simulink model "WPT_1"  (R2024a)
settings: Solver=VariableStepAuto  StartTime=0.0  StopTime=5  RelTol=1e-3
libraries: spsDiodeLib x9, spsSeriesRLCBranchLib x7, spsMosfetLib x5, spsVoltageMeasurementLib x4, spsCurrentMeasurementLib x3, spsMeanLib x3, spsACVoltageSourceLib x1, spsMutualInductanceLib x1, sps_lib x1
settings Model: Creator=Vivek Chadgal  LastModifiedBy=Vivek Chadgal
settings SolverCC: ZeroCrossAlgorithm=Adaptive
settings DebuggingCC: IgnoredZcDiagnostic=none

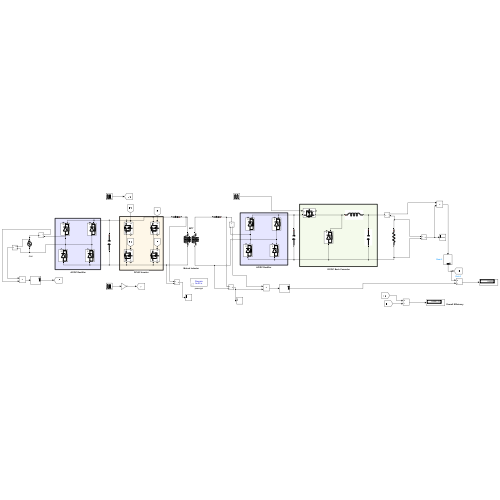
[thumbnail: Simulink's stored preview of the top-level diagram]
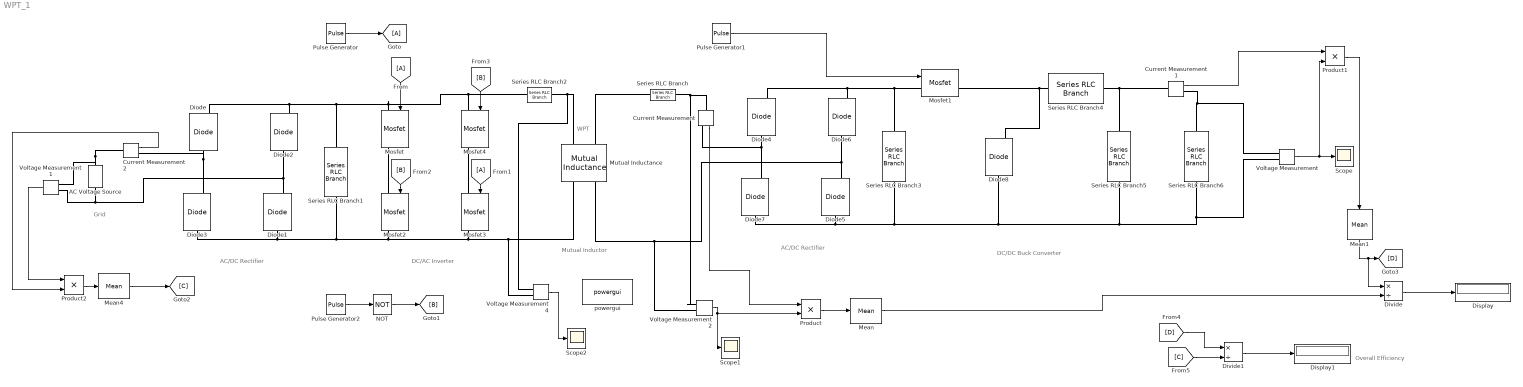
== system WPT_1 ==
  note: Overall Efficiency
  note: WPT
  note: Mutual Inductor
  note: Grid
  note: AC/DC Rectifier
  note: DC/DC Buck Converter
  note: DC/AC Inverter
  note: AC/DC Rectifier
  AC Voltage Source : spsACVoltageSourceLib/AC Voltage Source  Amplitude=230  Phase=0  Frequency=50  SampleTime=0  Measurements=None  BusType=swing  Pref=10e3  Qref=0  Qmin=-inf  Qmax=+inf
  Current Measurement : spsCurrentMeasurementLib/Current Measurement  PhasorSimulation=off  OutputType=Complex  PSBequivalent=0
  Current Measurement1 : spsCurrentMeasurementLib/Current Measurement  PhasorSimulation=off  OutputType=Complex  PSBequivalent=0
  Current Measurement2 : spsCurrentMeasurementLib/Current Measurement  PhasorSimulation=off  OutputType=Complex  PSBequivalent=0
  Diode{,1..8} (9 alike) : spsDiodeLib/Diode  Ron=0.001  Lon=0  Vf=0.8  IC=0  UseSnubber=0  Rs=500  Cs=250e-9  Measurements=on
  Display : Display
  Display1 : Display
  Divide : Product  Inputs=*/
  Divide1 : Product  Inputs=*/
  From : From
  From1 : From
  Goto : Goto
  Mean : spsMeanLib/Mean  Freq=50  Vinit=0  Ts=0
  Mean1 : spsMeanLib/Mean  Freq=50  Vinit=0  Ts=0
  Mean4 : spsMeanLib/Mean  Freq=50  Vinit=0  Ts=0
  Mosfet{,1..4} (5 alike) : spsMosfetLib/Mosfet  Ron=0.1  Lon=0  Rd=0.01  Vfd=0  IC=0  Rs=1e5  Cs=inf  Measurements=on
  Mutual Inductance : spsMutualInductanceLib/Mutual Inductance  LConnTagsString=a|b  RConnTagsString=A|B  TypeOfMutual=Two or three windings with equal mutual terms  NumberOfWindings=2  SelfImpedance1=[0 0.25]  SelfImpedance2=[ 0 0.25]  ThreeWindings=off  SelfImpedance3=[ 1.1 1.1e-03]  MutualImpedance=[0 0.125]  InductanceMatrix="[1.0 0.9  0.9 ;  0.9 1.0  0.9;  0.9 0.9 1.0 ] * 1e-3"  ResistanceMatrix="[1.0 0.9  0.9 ;  0.9 1.0  0.9;  0.9 0.9 1.0 ]"  Measurements=Winding voltages and currents
      settings: LibrarySourceBlock=sps_lib/Passives/Mutual Inductance
  NOT : Logic  Operator=NOT  IconShape=distinctive  AllPortsSameDT=off  OutDataTypeStr=boolean
  Product : Product
  Product1 : Product
  Product2 : Product
  Pulse Generator : DiscretePulseGenerator  PulseType=Time based  Amplitude=5  Period=0.02  PulseWidth=50
  Pulse Generator1 : DiscretePulseGenerator  PulseType=Time based  Amplitude=5  Period=0.02  PulseWidth=50
  Pulse Generator2 : DiscretePulseGenerator  PulseType=Time based  Amplitude=50  Period=0.02  PulseWidth=5
  Scope : Scope
  Scope1 : Scope
  Scope2 : Scope
  Series RLC Branch : spsSeriesRLCBranchLib/Series RLC Branch  LConnTagsString=__new0  RConnTagsString=__new0  BranchType=C  Resistance=1  Inductance=1e-3  SetiL0=off  InitialCurrent=0  Capacitance=4.691e-6  Setx0=off  InitialVoltage=0  Measurements=None
  Series RLC Branch1 : spsSeriesRLCBranchLib/Series RLC Branch  LConnTagsString=__new0  RConnTagsString=__new0  BranchType=C  Resistance=1  Inductance=1e-3  SetiL0=off  InitialCurrent=0  Capacitance=10e-6  Setx0=off  InitialVoltage=0  Measurements=None
  Series RLC Branch2 : spsSeriesRLCBranchLib/Series RLC Branch  LConnTagsString=__new0  RConnTagsString=__new0  BranchType=C  Resistance=1  Inductance=1e-3  SetiL0=off  InitialCurrent=0  Capacitance=4.691e-6  Setx0=off  InitialVoltage=0  Measurements=None
  Series RLC Branch3 : spsSeriesRLCBranchLib/Series RLC Branch  LConnTagsString=__new0  RConnTagsString=__new0  BranchType=C  Resistance=1  Inductance=1e-3  SetiL0=off  InitialCurrent=0  Capacitance=1000e-6  Setx0=off  InitialVoltage=0  Measurements=None
  Series RLC Branch4 : spsSeriesRLCBranchLib/Series RLC Branch  LConnTagsString=__new0  RConnTagsString=__new0  BranchType=L  Resistance=1  Inductance=1e-3  SetiL0=off  InitialCurrent=0  Capacitance=1e-6  Setx0=off  InitialVoltage=0  Measurements=None
  Series RLC Branch5 : spsSeriesRLCBranchLib/Series RLC Branch  LConnTagsString=__new0  RConnTagsString=__new0  BranchType=C  Resistance=1  Inductance=1e-3  SetiL0=off  InitialCurrent=0  Capacitance=1000e-6  Setx0=off  InitialVoltage=0  Measurements=None
  Series RLC Branch6 : spsSeriesRLCBranchLib/Series RLC Branch  LConnTagsString=__new0  RConnTagsString=__new0  BranchType=R  Resistance=1000  Inductance=1e-3  SetiL0=off  InitialCurrent=0  Capacitance=1e-6  Setx0=off  InitialVoltage=0  Measurements=None
  Voltage Measurement{,1..2,4} (4 alike) : spsVoltageMeasurementLib/Voltage Measurement  PhasorSimulation=off  OutputType=Complex  PSBequivalent=0
  powergui : sps_lib/powergui  Priority=1  SimulationMode=Discrete  SampleTime=50e-6  frequency=60  Iterations=50  frequencyindice=50  Pbase=100e6  ErrMax=1e-4  UnitsV=kV  UnitsW=MW  buscounter=0  FunctionMessages=off  echomessages=off  EnableUseOfTLC=off  CurrentSourceSwitches=off  DisableSnubberDevices=off  DisableRonSwitches=off  DisableVfSwitches=off  DisplayEquations=off  AutomaticDiscreteSolvers=off  SolverType=Tustin/Backward Euler (TBE)  Interpol=off  ExternalGateDelay=off  methode=off  Ts=100  x0status=blocks  SPID=on  SwTol=0  HookPort=off  NonlinearTolerance=1e-4  nMaxIteration=100  ContinueOnMaxIteration=off  RestoreLinks=warning  ResistiveCurrentMeasurement=off  Frange=[0:2:500]  Ylog=off  Xlog=on  ShowGrid=off  save=off  variable=ZData  structure=0  ZoomFFT=off  StartTime=0.0  cycles=1  DisplayStyle=1  fundamental=60  FreqAxis=off  MaxFrequency=1000  frequencyindicesteady=1  RmsSteady=1  display=off
  wires:
  Pulse Generator/1 -> Goto/1
  From/1 -> Mosfet/1
  From1/1 -> Mosfet3/1
  [B] -> Mosfet2/1
  [B] -> Mosfet4/1
  Pulse Generator2/1 -> NOT/1
  NOT/1 -> [B]
  Pulse Generator1/1 -> Mosfet1/1
  Voltage Measurement/1 -> Product1/2, Scope/1
  Voltage Measurement2/1 -> Scope1/1, Product/2
  Voltage Measurement4/1 -> Scope2/1
  Current Measurement/1 -> Product/1
  Current Measurement1/1 -> Product1/1
  Product/1 -> Mean/1
  Divide/1 -> Display/1
  Mean/1 -> Divide/2
  Product1/1 -> Mean1/1
  Product2/1 -> Mean4/1
  Divide1/1 -> Display1/1
  [D] -> Divide1/1
  [C] -> Divide1/2
  Current Measurement2/1 -> Product2/2
  Voltage Measurement1/1 -> Product2/1
  Mean4/1 -> [C]
  Mean1/1 -> [D], Divide/1
  connections:
  Diode/LConn1 -- Diode3/RConn1 -- Current Measurement2/RConn1
  Diode2/LConn1 -- Voltage Measurement1/LConn2 -- AC Voltage Source/LConn1 -- Diode1/RConn1
  Mosfet2/LConn1 -- Mosfet/RConn1
  Mosfet4/RConn1 -- Mosfet3/LConn1
  Diode/RConn1 -- Mosfet/LConn1 -- Series RLC Branch2/RConn1 -- Mosfet4/LConn1 -- Series RLC Branch1/LConn1 -- Diode2/RConn1
  Diode3/LConn1 -- Mosfet2/RConn1 -- Voltage Measurement4/LConn2 -- Mutual Inductance/RConn1 -- Mosfet3/RConn1 -- Series RLC Branch1/RConn1 -- Diode1/LConn1
  Series RLC Branch2/LConn1 -- Voltage Measurement4/LConn1 -- Mutual Inductance/LConn1
  Mutual Inductance/LConn2 -- Series RLC Branch/RConn1
  Voltage Measurement2/LConn1 -- Current Measurement/LConn1 -- Series RLC Branch/LConn1
  Diode7/LConn1 -- Voltage Measurement/LConn2 -- Series RLC Branch6/RConn1 -- Series RLC Branch5/RConn1 -- Diode8/LConn1 -- Series RLC Branch3/RConn1 -- Diode5/LConn1
  Diode6/LConn1 -- Voltage Measurement2/LConn2 -- Mutual Inductance/RConn2 -- Diode5/RConn1
  Diode6/RConn1 -- Mosfet1/LConn1 -- Series RLC Branch3/LConn1 -- Diode4/RConn1
  Series RLC Branch4/LConn1 -- Diode8/RConn1 -- Mosfet1/RConn1
  Series RLC Branch4/RConn1 -- Current Measurement1/LConn1 -- Series RLC Branch5/LConn1
  Diode4/LConn1 -- Current Measurement/RConn1 -- Diode7/RConn1
  Series RLC Branch6/LConn1 -- Current Measurement1/RConn1 -- Voltage Measurement/LConn1
  AC Voltage Source/RConn1 -- Voltage Measurement1/LConn1 -- Current Measurement2/LConn1
